simulink model "EXE2"  (R2019b)
settings: Solver=VariableStepAuto  StartTime=0.0  StopTime=0.06  RelTol=1e-3
libraries: powerlib x22, powerlib_meascontrol x4
settings Model: Creator=DELL  LastModifiedBy=96547
settings DataIOCC: InspectSignalLogs=on

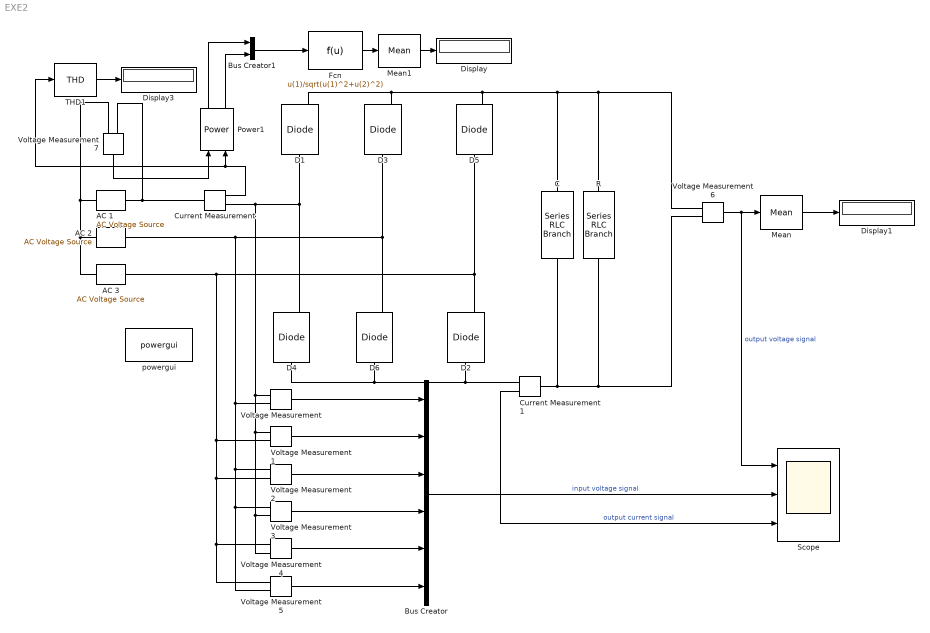
== system EXE2 ==
  " C" : powerlib/Elements/Series RLC Branch  LConnTagsString=__new0  RConnTagsString=__new0  BranchType=C  Resistance=1  Inductance=5e-3  SetiL0=off  InitialCurrent=0  Capacitance=5.5e-3  Setx0=off  InitialVoltage=0  Measurements=None
      settings: SourceProductName=Simscape Electrical
  " R" : powerlib/Elements/Series RLC Branch  LConnTagsString=__new0  RConnTagsString=__new0  BranchType=R  Resistance=1  Inductance=5e-3  SetiL0=off  InitialCurrent=0  Capacitance=0  Setx0=off  InitialVoltage=0  Measurements=None
      settings: SourceProductName=Simscape Electrical
  "AC 1 " : powerlib/Electrical Sources/AC Voltage Source  Amplitude=310  Phase=0  Frequency=50  SampleTime=0  Measurements=None  BusType=swing  Pref=10e3  Qref=0  Qmin=-inf  Qmax=+inf
      settings: SourceProductName=Simscape Electrical
  AC 2 : powerlib/Electrical Sources/AC Voltage Source  Amplitude=310  Phase=-120  Frequency=50  SampleTime=0  Measurements=None  BusType=swing  Pref=10e3  Qref=0  Qmin=-inf  Qmax=+inf
      settings: SourceProductName=Simscape Electrical
  AC 3 : powerlib/Electrical Sources/AC Voltage Source  Amplitude=310  Phase=-240  Frequency=50  SampleTime=0  Measurements=None  BusType=swing  Pref=10e3  Qref=0  Qmin=-inf  Qmax=+inf
      settings: SourceProductName=Simscape Electrical
  Bus Creator : BusCreator  Inputs=6
  Bus Creator1 : BusCreator  Inputs=2
  Current Measurement : powerlib/Measurements/Current Measurement  PhasorSimulation=off  OutputType=Complex  PSBequivalent=0
      settings: SourceProductName=Simscape Electrical
  Current Measurement1 : powerlib/Measurements/Current Measurement  PhasorSimulation=off  OutputType=Complex  PSBequivalent=0
      settings: SourceProductName=Simscape Electrical
  D{1..6} (6 alike) : powerlib/Power Electronics/Diode  Ron=0.001  Lon=0  Vf=0.8  IC=0  UseSnubber=0  Rs=500  Cs=250e-9  Measurements=on
      settings: SourceProductName=Simscape Electrical
  Display : Display
  Display1 : Display
  Display3 : Display
  Fcn : Fcn  Expr=u(1)/sqrt(u(1)^2+u(2)^2)
  Mean : powerlib_meascontrol/Measurements/Mean  Freq=60  Vinit=0  Ts=0
      settings: SourceProductName=Simscape Electrical
  Mean1 : powerlib_meascontrol/Measurements/Mean  Freq=60  Vinit=0  Ts=0
      settings: SourceProductName=Simscape Electrical
  Power1 : powerlib_meascontrol/Measurements/Power  Freq=50  Vinit=[1, 0]  Iinit=[1, 0]  Ts=0
      settings: SourceProductName=Simscape Electrical
  Scope : Scope  NumInputPorts=3
  THD1 : powerlib_meascontrol/Measurements/THD  Freq=50  Ts=0
      settings: SourceProductName=Simscape Electrical
  Voltage Measurement{,1..7} (8 alike) : powerlib/Measurements/Voltage Measurement  PhasorSimulation=off  OutputType=Complex  PSBequivalent=0
      settings: SourceProductName=Simscape Electrical
  powergui : powerlib/powergui  Priority=1  SimulationMode=Continuous  SampleTime=50e-6  frequency=60  Iterations=50  frequencyindice=50  Pbase=100e6  ErrMax=1e-4  UnitsV=kV  UnitsW=MW  buscounter=0  FunctionMessages=off  echomessages=off  EnableUseOfTLC=off  CurrentSourceSwitches=off  DisableSnubberDevices=off  DisableRonSwitches=off  DisableVfSwitches=off  DisplayEquations=off  AutomaticDiscreteSolvers=off  SolverType=Tustin/Backward Euler (TBE)  Interpol=off  ExternalGateDelay=off  methode=off  Ts=100  x0status=blocks  SPID=on  SwTol=0  HookPort=off  NonlinearTolerance=1e-4  nMaxIteration=100  ContinueOnMaxIteration=off  RestoreLinks=warning  ResistiveCurrentMeasurement=off  Frange=[0:2:500]  Ylog=off  Xlog=on  ShowGrid=off  save=off  variable=ZData  structure=0  ZoomFFT=off  StartTime=0.0  cycles=1  DisplayStyle=1  fundamental=60  FreqAxis=off  MaxFrequency=1000  frequencyindicesteady=1  RmsSteady=1  display=off
      settings: SourceProductName=Simscape Electrical
  wires:
  Voltage Measurement/1 -> Bus Creator/1
  Voltage Measurement1/1 -> Bus Creator/2
  Voltage Measurement2/1 -> Bus Creator/3
  Voltage Measurement3/1 -> Bus Creator/4
  Voltage Measurement4/1 -> Bus Creator/5
  Voltage Measurement5/1 -> Bus Creator/6
  Voltage Measurement6/1 -> Scope/1, Mean/1  "output voltage signal"
  Bus Creator1/1 -> Fcn/1
  Mean/1 -> Display1/1
  Voltage Measurement7/1 -> Power1/1
  Current Measurement/1 -> THD1/1, Power1/2
  Power1/1 -> Bus Creator1/1
  Power1/2 -> Bus Creator1/2
  THD1/1 -> Display3/1
  Fcn/1 -> Mean1/1
  Mean1/1 -> Display/1
  Current Measurement1/1 -> Scope/3  "output current signal"
  Bus Creator/1 -> Scope/2  "input voltage signal"
  connections:
  Voltage Measurement4/LConn2 -- Voltage Measurement3/LConn2 -- Voltage Measurement1/LConn1 -- Voltage Measurement/LConn1 -- D1/LConn1 -- D4/RConn1 -- Current Measurement/RConn1
  Voltage Measurement/LConn2 -- Voltage Measurement2/LConn1 -- Voltage Measurement5/LConn2 -- Voltage Measurement3/LConn1 -- D6/RConn1 -- D3/LConn1 -- AC 2/RConn1
  Voltage Measurement5/LConn1 -- Voltage Measurement4/LConn1 -- Voltage Measurement2/LConn2 -- Voltage Measurement1/LConn2 -- D2/RConn1 -- D5/LConn1 -- AC 3/RConn1
  D1/RConn1 -- D3/RConn1 -- D5/RConn1 -- Voltage Measurement6/LConn1 -- " R"/LConn1 -- " C"/LConn1
  " C"/RConn1 -- Current Measurement1/LConn1 -- Voltage Measurement6/LConn2 -- " R"/RConn1
  "AC 1 "/LConn1 -- Voltage Measurement7/LConn2 -- AC 2/LConn1 -- AC 3/LConn1
  Current Measurement/LConn1 -- Voltage Measurement7/LConn1 -- "AC 1 "/RConn1
  D2/LConn1 -- Current Measurement1/RConn1 -- D6/LConn1 -- D4/LConn1
